simulink library "CrossProdMatrix_lib"  (R2018b)
settings: Solver=VariableStepAuto  StartTime=0.0  StopTime=10.0  RelTol=1e-3
libraries: sharedutil x1
settings Model: Creator=kylle  LastModifiedBy=Taylor

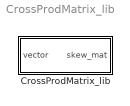
== system CrossProdMatrix_lib ==
  CrossProdMatrix_lib : Subsystem  TreatAsAtomicUnit=on
      settings: RTWFcnNameOpts=Use subsystem name  RTWFileNameOpts=Use subsystem name

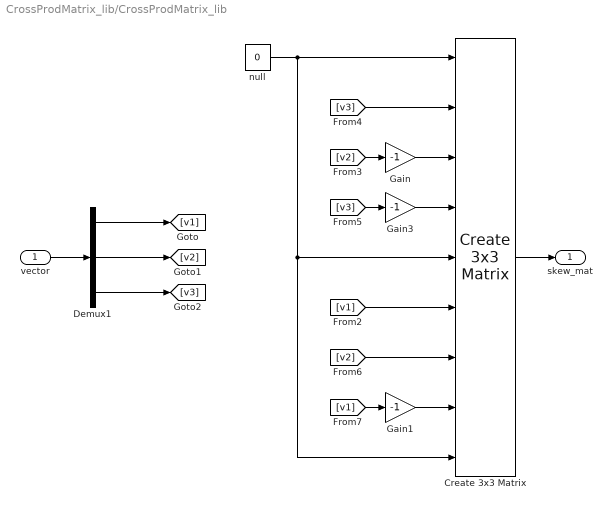
== system CrossProdMatrix_lib/CrossProdMatrix_lib ==
  vector : Inport
  Create 3x3 Matrix : sharedutil/Create 3x3 Matrix  aMode=aMode
  Demux1 : Demux  Outputs=3
  Gain : Gain  Gain=-1
  Gain1 : Gain  Gain=-1
  Gain3 : Gain  Gain=-1
  null : Constant  Value=0
  skew_mat : Outport
  wires:
  Gain3/1 -> Create 3x3 Matrix/4
  null/1 -> Create 3x3 Matrix/9, Create 3x3 Matrix/5, Create 3x3 Matrix/1
  Create 3x3 Matrix/1 -> skew_mat/1
  Gain/1 -> Create 3x3 Matrix/3
  Demux1/2 -> [v2]
  Demux1/1 -> [v1]
  [v1] -> Gain1/1
  [v3] -> Create 3x3 Matrix/2
  [v2] -> Create 3x3 Matrix/7
  Demux1/3 -> [v3]
  [v3] -> Gain3/1
  [v1] -> Create 3x3 Matrix/6
  Gain1/1 -> Create 3x3 Matrix/8
  vector/1 -> Demux1/1
  [v2] -> Gain/1
